simulink model "p4amodel"  (Simulink 8.7)
settings: Solver=FixedStepAuto  SolverMode=SingleTasking  StartTime=0.0  StopTime=15.0  FixedStep=0.2  RelTol=1e-3
settings Model: Creator=eispin  LastModifiedBy=eispin
settings DataIOCC: SaveFormat=Dataset  SaveOutput=off  SaveTime=off
settings OptimizationCC: BlockReduction=off  BooleanDataType=off
settings DebuggingCC: SaveWithParameterizedLinksMsg=none  SignalResolutionControl=TryResolveAllWithWarning  AllowSymbolicDim=off
settings HardwareCC: ProdBitPerPointer=64  ProdLargestAtomicFloat=Float  ProdIntDivRoundTo=Zero  ProdEndianess=LittleEndian  ProdWordSize=64  ProdHWDeviceType=Intel->x86-64 (Windows64)  TargetUnknown=on
settings ModelReferenceCC: PropagateSignalLabelsOutOfModel=on
settings ConfigComp: CovModelRefEnable=off

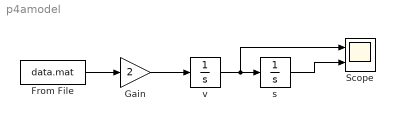
== system p4amodel ==
  From File : FromFile  FileName=data.mat  SampleTime=0  InterpolationWithinTimeRange=Zero order hold
  Gain : Gain  Gain=2
  Scope : Scope  NumInputPorts=2
  s : Integrator
  v : Integrator
  wires:
  From File/1 -> Gain/1
  Gain/1 -> v/1
  s/1 -> Scope/2
  v/1 -> s/1, Scope/1
